simulink model "Pulsformung"  (Simulink 7.8)
settings: Solver=FixedStepDiscrete  StartTime=0  StopTime=1e5  RelTol=1e-3
undefined symbols (not defined in the file or in its folder): Fs, sided, Two
libraries: dspsnks4 x4, commdigbbndam3 x1, simulink x1, commrandsrc2 x1, commfilt2 x1, dspsigops x1, dspsrcs4 x1
settings Model: Creator=schwall  LastModifiedBy=schwall
settings DataIOCC: SaveOutput=off  SignalLogging=off  SaveTime=off
settings DebuggingCC: FcnCallInpInsideContextMsg=Use local settings  StrictBusMsg=Warning

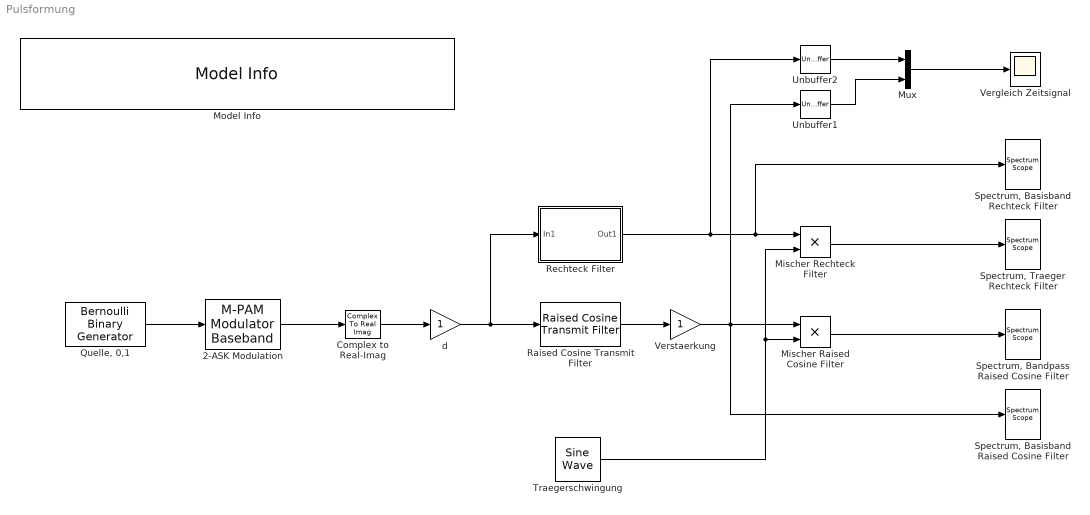
== system Pulsformung ==
  2-ASK Modulation : commdigbbndam3/M-PAM Modulator Baseband  M=2  InType=Integer  Enc=Binary  PowType=Min. distance between symbols  MinDist=2  AvgPow=1  PeakPow=1  outDtype=double  outWordLen=16  outUDDataType=sfix(16)  outFracLenMode=Best precision  outFracLen=15
  Complex to Real-Imag : ComplexToRealImag  Output=Real
  Mischer Raised Cosine Filter : Product  RndMeth=Zero
  Mischer Rechteck Filter : Product  RndMeth=Zero
  Model Info : simulink/Model-Wide Utilities/Model Info  InitialBlockCM=None  BlockCM=None  Frame=on  DisplayStringWithTags=|  HorizontalTextAlignment=Left  LeftAlignmentValue=0.02  SourceBlockDiagram=Pulsformung  TagMaxNumber=20
      | Demo Pulsformung
      | Vorlesung Nachrichtentechnik II
      | Institut für Nachrichtentechnik (CEL)
  Mux : Mux  Inputs=2
  "Quelle, 0,1" : commrandsrc2/Bernoulli Binary Generator  P=0.5  seed=61  Ts=1/1000  frameBased=on  sampPerFrame=8  orient=off  outDataType=double
  Raised Cosine Transmit Filter : commfilt2/Raised Cosine Transmit Filter  filtType=Normal  D=4  R=0  sampMode=Mute  saveAsFlag=0  N=8  framing=Maintain input frame rate  InputProcessing=Columns as channels (frame based)  checkGain=User-specified  filterGain=1  checkCoeff=off  variableName=rcTxFilt  launchFVT=off  roundingMode=Floor  overflowMode=off
  Rechteck Filter : Subsystem
      mask Display: plot([zeros(1,64) ones(1,128) zeros(1,64)])
  "Spectrum, Bandpass Raised Cosine Filter" : dspsnks4/Spectrum Scope  ScopeProperties=on  Domain=Frequency  HorizSpan=1  UseBuffer=off  BufferSize=128  Overlap=64  TreatMby1Signals=One channel  inpFftLenInherit=on  FFTlength=128  numAvg=25  DisplayProperties=off  AxisGrid=on  Memory=off  FrameNumber=on  AxisLegend=off  AxisZoom=off  OpenScopeAtSimStart=on  OpenScopeImmediately=off  FigPos=[561 43 426 247]  AxisProperties=off  XUnits=Hertz  XRange=Two-sided ((-Fs/2...Fs/2])  XDisplay=0  InheritXIncr=on  XIncr=1.0  XLabel=Samples  XLimit=User-defined  YUnits=dBW/Hertz  XMax=4000  XMin=-4000  YLabel=Magnitude-squared, dB  LineProperties=off  LineColors=[1 0 0]  wintypeSpecScope=Hann  RsSpecScope=50  betaSpecScope=5  winsampSpecScope=Periodic  XAxisParamsVer=6.9  isFrameUpgraded=on
      settings: YMin=-91.6959  YMax=-32.354
  "Spectrum, Basisband Raised Cosine Filter" : dspsnks4/Spectrum Scope  ScopeProperties=on  Domain=Frequency  HorizSpan=1  UseBuffer=off  BufferSize=128  Overlap=64  TreatMby1Signals=One channel  inpFftLenInherit=on  FFTlength=128  numAvg=25  DisplayProperties=off  AxisGrid=on  Memory=off  FrameNumber=on  AxisLegend=off  AxisZoom=off  OpenScopeAtSimStart=on  OpenScopeImmediately=off  FigPos=[560 387 422 298]  AxisProperties=off  XUnits=Hertz  XRange=Two-sided ((-Fs/2...Fs/2])  XDisplay=0  InheritXIncr=on  XIncr=1.0  XLabel=Samples  XLimit=User-defined  YUnits=dBW/Hertz  XMax=4000  XMin=-4000  YLabel=Magnitude-squared, dB  LineProperties=off  LineColors=[0 0 1]  wintypeSpecScope=Hann  RsSpecScope=50  betaSpecScope=5  winsampSpecScope=Periodic  XAxisParamsVer=6.9  isFrameUpgraded=on
      settings: YMin=-92.1934  YMax=-20
  "Spectrum, Basisband Rechteck Filter" : dspsnks4/Spectrum Scope  ScopeProperties=on  Domain=Frequency  HorizSpan=1  UseBuffer=off  BufferSize=128  Overlap=64  TreatMby1Signals=One channel  inpFftLenInherit=on  FFTlength=128  numAvg=25  DisplayProperties=off  AxisGrid=on  Memory=off  FrameNumber=on  AxisLegend=off  AxisZoom=off  OpenScopeAtSimStart=on  OpenScopeImmediately=off  FigPos=[46 388 495 297]  AxisProperties=off  XUnits=Hertz  XRange=Two-sided ((-Fs/2...Fs/2])  XDisplay=0  InheritXIncr=on  XIncr=1.0  XLabel=Samples  XLimit=User-defined  YUnits=dBW/Hertz  XMax=4000  XMin=-4000  YLabel=Magnitude-squared, dB  LineProperties=off  LineColors=[0 0 1]  wintypeSpecScope=Hann  RsSpecScope=50  betaSpecScope=5  winsampSpecScope=Periodic  XAxisParamsVer=6.9  isFrameUpgraded=on
      settings: YMin=-63.0637  YMax=-20
  "Spectrum, Traeger Rechteck Filter" : dspsnks4/Spectrum Scope  ScopeProperties=on  Domain=Frequency  HorizSpan=1  UseBuffer=off  BufferSize=128  Overlap=64  TreatMby1Signals=One channel  inpFftLenInherit=on  FFTlength=128  numAvg=25  DisplayProperties=off  AxisGrid=on  Memory=off  FrameNumber=on  AxisLegend=off  AxisZoom=off  OpenScopeAtSimStart=on  OpenScopeImmediately=off  FigPos=[44 40 496 252]  AxisProperties=off  XUnits=Hertz  XRange=Two-sided ((-Fs/2...Fs/2])  XDisplay=0  InheritXIncr=on  XIncr=1.0  XLabel=Samples  XLimit=User-defined  YUnits=dBW/Hertz  XMax=4000  XMin=-4000  YLabel=Magnitude-squared, dB  LineProperties=off  LineColors=[1 0 0]  wintypeSpecScope=Hann  RsSpecScope=50  betaSpecScope=5  winsampSpecScope=Periodic  XAxisParamsVer=6.9  isFrameUpgraded=on
      settings: YMin=-88.4081  YMax=-31.6208
  Traegerschwingung : dspsrcs4/Sine Wave  Amplitude=1  Frequency=2000  Phase=pi/4  SampleMode=Discrete  OutComplex=Real  CompMethod=Trigonometric fcn  TableSize=Speed  SampleTime=1/8000  SamplesPerFrame=64  ResetState=Restart at time zero  dataType=double  wordLen=16  udDataType=sfix(16)  fracBitsMode=Best precision  numFracBits=15  OutDataTypeStr=double  LastOutDataTypeStr=double
  Unbuffer1 : Unbuffer
  Unbuffer2 : Unbuffer
  Vergleich Zeitsignal : Scope
      settings: YMin=-4  YMax=4  SaveName=ScopeData2
  Verstaerkung : Gain
  d : Gain
  wires:
  "Quelle, 0,1"/1 -> 2-ASK Modulation/1
  2-ASK Modulation/1 -> Complex to Real-Imag/1
  Complex to Real-Imag/1 -> d/1
  d/1 -> Raised Cosine Transmit Filter/1, Rechteck Filter/1(In1)
  Raised Cosine Transmit Filter/1 -> Verstaerkung/1
  Mux/1 -> Vergleich Zeitsignal/1
  Unbuffer2/1 -> Mux/1
  Rechteck Filter/1(Out1) -> Unbuffer2/1, Mischer Rechteck Filter/1, "Spectrum, Basisband Rechteck Filter"/1
  Verstaerkung/1 -> Unbuffer1/1, Mischer Raised Cosine Filter/1, "Spectrum, Basisband Raised Cosine Filter"/1
  Unbuffer1/1 -> Mux/2
  Mischer Rechteck Filter/1 -> "Spectrum, Traeger Rechteck Filter"/1
  Mischer Raised Cosine Filter/1 -> "Spectrum, Bandpass Raised Cosine Filter"/1
  Traegerschwingung/1 -> Mischer Raised Cosine Filter/2, Mischer Rechteck Filter/2

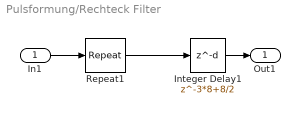
== system Pulsformung/Rechteck Filter ==
  In1 : Inport
  Integer Delay1 : Delay  DelayLength=3*8+8/2  InputProcessing=Inherited
  Repeat1 : dspsigops/Repeat  N=8  InputProcessing=Inherited (this choice will be removed - see release notes)  RateOptions=Enforce single-rate processing  ic=0  mode=Unused parameter value
  Out1 : Outport
  wires:
  Repeat1/1 -> Integer Delay1/1
  In1/1 -> Repeat1/1
  Integer Delay1/1 -> Out1/1
